simulink model "ModeInputHandle"  (R2018b)
settings: Solver=FixedStepDiscrete  StartTime=0.0  StopTime=10.0  FixedStep=0.01  RelTol=1e-3
undefined symbols (not defined in the file or in its folder): c, CmprtMdHMIReqExt2Tp1, CmprtMdHMIReqExtTp1, CmprtMdHMIReqTp1, d, e, EZESwReq1, f, g, IfVeSMSeStNumConfig, j, KeSMSuButtonLongPressedThrshldTm_Val, KeSMSuFoldType_Val, KeSMSwSeatSMSSeatMdTrigGapTimer_Val, KeSMSwSeatTrigWaitTimer_Val, KeSMSwSRSActiveValidTm_Val, LckUlckActvtFunc1, LstLckFunc1, LugSelectSw1, MdReqTp1, PowerMode1, SeatOccupiedSts1, SRSMode1, StPassCmprtMdCtrl_Md10_VCUConfig_Val, StPassCmprtMdCtrl_Md11_VCUConfig_Val, StPassCmprtMdCtrl_Md12_VCUConfig_Val, StPassCmprtMdCtrl_Md13_VCUConfig_Val, StPassCmprtMdCtrl_Md1_VCUConfig_Val, StPassCmprtMdCtrl_Md27_VCUConfig_Val, StPassCmprtMdCtrl_Md28_VCUConfig_Val, StPassCmprtMdCtrl_Md29_VCUConfig_Val, StPassCmprtMdCtrl_Md2_VCUConfig_Val, StPassCmprtMdCtrl_Md30_VCUConfig_Val, StPassCmprtMdCtrl_Md31_VCUConfig_Val, StPassCmprtMdCtrl_Md32_VCUConfig_Val, StPassCmprtMdCtrl_Md3_VCUConfig_Val, StPassCmprtMdCtrl_Md53_VCUConfig_Val, StPassCmprtMdCtrl_Md56_VCUConfig_Val, StPassCmprtMdCtrl_Md57_VCUConfig_Val, StPassCmprtMdCtrl_Md58_VCUConfig_Val, StPassCmprtMdCtrl_Md61_VCUConfig_Val, StPassCmprtMdCtrl_Md62_VCUConfig_Val, StPassCmprtMdCtrl_Md8_VCUConfig_Val, StPassCmprtMdCtrl_Md9_VCUConfig_Val, StSrv_StMd10_Config_Val, StSrv_StMd11_Config_Val, StSrv_StMd12_Config_Val, StSrv_StMd13_Config_Val, StSrv_StMd1_Config_Val, StSrv_StMd27_Config_Val, StSrv_StMd28_Config_Val, StSrv_StMd29_Config_Val, StSrv_StMd2_Config_Val, StSrv_StMd30_Config_Val, StSrv_StMd31_Config_Val, StSrv_StMd32_Config_Val, StSrv_StMd3_Config_Val, StSrv_StMd8_Config_Val, StSrv_StMd9_Config_Val, VehMovState1
libraries: MSMLib x91
(part 7 of 9)

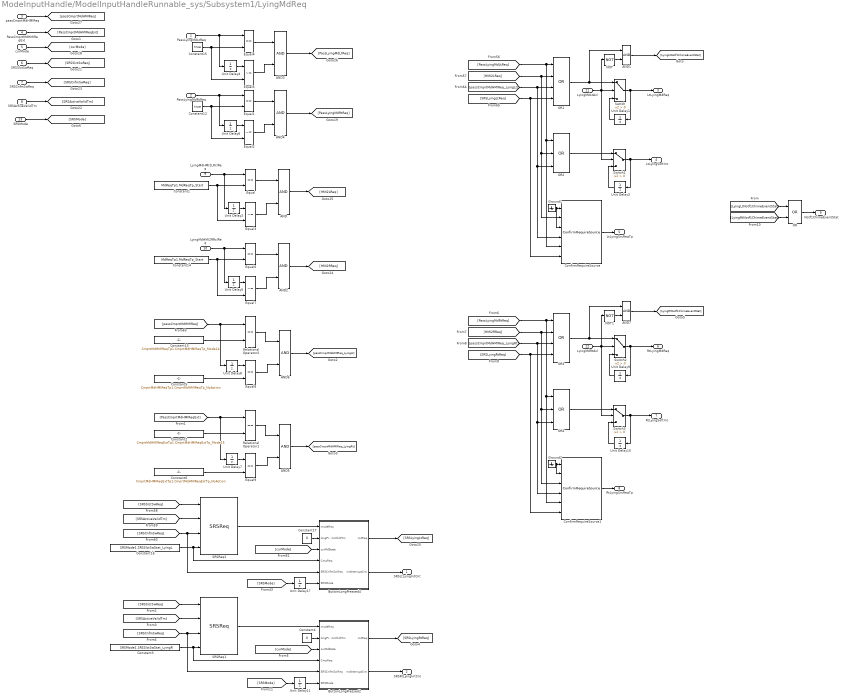
== system ModeInputHandle/ModelInputHandleRunnable_sys/Subsystem1/LyingMdReq ==
  PassLyingMdLtReq : Inport
  PassLyingMdRtReq : Inport  Port=2
  passCmprtMdHMIReq : Inport  Port=3
  PassCmprtMdHMIReqExt : Inport  Port=4
  curMode : Inport  Port=5
  SRSSlctSwReq : Inport  Port=6
  SRSCnfmSwReq : Inport  Port=7
  SRSActiveValidTm : Inport  Port=8
  LyingMdHMI2LRclReq : Inport  Port=9
  LyingMdHMI2RRclReq : Inport  Port=10
  LyingMdLtAvl : Inport  Port=11
  LyingMdRtAvl : Inport  Port=12
  SRSMode : Inport  Port=13
  AND{,1..7} (8 alike) : Logic  AllPortsSameDT=off  OutDataTypeStr=boolean
  ButtonLongPressed2 : Subsystem  AncestorBlock=MSMLib/ButtonLongPressed
  ButtonLongPressed4 : Subsystem  AncestorBlock=MSMLib/ButtonLongPressed
  ConfirmRequireSource : MSMLib/ConfirmRequireSource  SystemSampleTime=-1
  ConfirmRequireSource1 : MSMLib/ConfirmRequireSource  SystemSampleTime=-1
  Constant1 : Constant  Value=MdReqTp1.MdReqTp_Start
  Constant12 : Constant  Value=true  OutDataTypeStr=boolean
  Constant13 : Constant  Value=CmprtMdHMIReqTp1.CmprtMdHMIReqTp_Mode14  OutDataTypeStr=Enum:CmprtMdHMIReqTp1
  Constant14 : Constant  Value=MdReqTp1.MdReqTp_Start
  Constant15 : Constant  Value=true  OutDataTypeStr=boolean
  Constant16 : Constant  Value=SRSMode1.SRSSlctSwStat_LyingL  OutDataTypeStr=Enum:SRSMode1
  Constant17 : Constant  Value=0  OutDataTypeStr=uint8
  Constant2 : Constant  Value=CmprtMdHMIReqExtTp1.CmprtMdHMIReqExtTp_Mode15  OutDataTypeStr=Enum:CmprtMdHMIReqExtTp1
  Constant3 : Constant  Value=SRSMode1.SRSSlctSwStat_LyingR  OutDataTypeStr=Enum:SRSMode1
  Constant4 : Constant  Value=0  OutDataTypeStr=uint8
  Constant5 : Constant  Value=CmprtMdHMIReqTp1.CmprtMdHMIReqTp_NoAction  OutDataTypeStr=Enum:CmprtMdHMIReqTp1
  Constant6 : Constant  Value=CmprtMdHMIReqExtTp1.CmprtMdHMIReqExtTp_NoAction  OutDataTypeStr=Enum:CmprtMdHMIReqExtTp1
  Equal{,1,4,6,8..9} (6 alike) : RelationalOperator  Operator===  OutDataTypeStr=boolean  RndMeth=Simplest
  Equal{2..3,5,7} (4 alike) : RelationalOperator  Operator=~=  OutDataTypeStr=boolean  RndMeth=Simplest
  Ground1 : Ground
  Ground2 : Ground
  NOT : Logic  Operator=NOT  AllPortsSameDT=off  OutDataTypeStr=boolean
  NOT1 : Logic  Operator=NOT  AllPortsSameDT=off  OutDataTypeStr=boolean
  OR : Logic  Operator=OR  AllPortsSameDT=off  OutDataTypeStr=boolean
  OR1 : Logic  Operator=OR  Inputs=4  AllPortsSameDT=off  OutDataTypeStr=boolean
  OR2 : Logic  Operator=OR  Inputs=3  AllPortsSameDT=off  OutDataTypeStr=boolean
  OR3 : Logic  Operator=OR  Inputs=4  AllPortsSameDT=off  OutDataTypeStr=boolean
  OR4 : Logic  Operator=OR  Inputs=3  AllPortsSameDT=off  OutDataTypeStr=boolean
  Relational Operator1 : RelationalOperator  Operator===  OutDataTypeStr=boolean  RndMeth=Simplest
  Relational Operator2 : RelationalOperator  Operator===  OutDataTypeStr=boolean  RndMeth=Simplest
  SRSReq1 : MSMLib/SRSReq  SystemSampleTime=-1
  SRSReq2 : MSMLib/SRSReq  SystemSampleTime=-1
  Switch{,1..3} (4 alike) : Switch  Criteria=u2 > Threshold
  Unit Delay{1,3..4,6,9..10} (6 alike) : UnitDelay  SampleTime=-1
  Unit Delay11 : UnitDelay  InitialCondition=d  SampleTime=-1
  Unit Delay17 : UnitDelay  InitialCondition=d  SampleTime=-1
  Unit Delay2 : UnitDelay  InitialCondition=e  SampleTime=-1
  Unit Delay5 : UnitDelay  InitialCondition=e  SampleTime=-1
  Unit Delay7 : UnitDelay  InitialCondition=g  SampleTime=-1
  Unit Delay8 : UnitDelay  InitialCondition=c  SampleTime=-1
  SRSLtLyingIntCnt : Outport
  SRSRtLyingIntCnt : Outport  Port=2
  LtLyingMdReq : Outport  Port=3
  LtLyingSoftInt : Outport  Port=4
  LtLyingSrcReqTp : Outport  Port=5
  RtLyingMdReq : Outport  Port=6
  RtLyingSoftInt : Outport  Port=7
  RtLyingSrcReqTp : Outport  Port=8
  Notf1ChimeEventStat : Outport  Port=9
  wires:
  Constant15/1 -> Equal4/2, Equal5/2
  Equal5/1 -> AND3/2
  PassLyingMdLtReq/1 -> Unit Delay4/1, Equal4/1
  Equal2/1 -> AND4/2
  Constant12/1 -> Equal1/2, Equal2/2
  AND4/1 -> [PassLyingMdRtReq]
  Unit Delay4/1 -> Equal5/1
  Equal1/1 -> AND4/1
  PassLyingMdRtReq/1 -> Unit Delay6/1, Equal1/1
  Equal4/1 -> AND3/1
  AND3/1 -> [PassLyingMdLtReq]
  Unit Delay6/1 -> Equal2/1
  passCmprtMdHMIReq/1 -> [passCmprtMdHMIReq]
  SRSActiveValidTm/1 -> [SRSActiveValidTm]
  SRSSlctSwReq/1 -> [SRSSlctSwReq]
  SRSCnfmSwReq/1 -> [SRSCnfmSwReq]
  curMode/1 -> [curMode]
  PassCmprtMdHMIReqExt/1 -> [PassCmprtMdHMIReqExt]
  AND/1 -> [HMI2LReq]
  Equal3/1 -> AND/2
  Equal/1 -> AND/1
  Equal6/1 -> AND2/1
  Constant1/1 -> Equal3/2, Equal/2
  Constant14/1 -> Equal7/2, Equal6/2
  AND2/1 -> [HMI2RReq]
  Equal7/1 -> AND2/2
  Unit Delay5/1 -> Equal7/1
  LyingMdHMI2RRclReq/1 -> Unit Delay5/1, Equal6/1
  Unit Delay2/1 -> Equal3/1
  LyingMdHMI2LRclReq/1 -> Unit Delay2/1, Equal/1
  Unit Delay7/1 -> Equal9/1
  AND5/1 -> [passCmprtMdHMIReq_LyingRt]
  Equal9/1 -> AND5/2
  [PassCmprtMdHMIReqExt] -> Unit Delay7/1, Relational Operator1/1
  Constant2/1 -> Relational Operator1/2
  Relational Operator1/1 -> AND5/1
  [passCmprtMdHMIReq] -> Unit Delay8/1, Relational Operator2/1
  Relational Operator2/1 -> AND6/1
  Equal8/1 -> AND6/2
  Constant13/1 -> Relational Operator2/2
  Unit Delay8/1 -> Equal8/1
  AND6/1 -> [passCmprtMdHMIReq_LyingLt]
  Constant3/1 -> ButtonLongPressed2/4(CmpReq), SRSReq1/4
  ButtonLongPressed2/1(mdReq) -> [SRSLyingRtReq]
  [SRSCnfmSwReq] -> ButtonLongPressed2/5(SRSCnfmSwReq), SRSReq1/3
  Constant4/1 -> ButtonLongPressed2/2(longPressThrshhldTm)
  [SRSSlctSwReq] -> SRSReq1/1
  ButtonLongPressed2/2(mdInterruptCnt) -> SRSRtLyingIntCnt/1
  SRSReq1/1 -> ButtonLongPressed2/1(modeReq)
  SRSReq2/1 -> ButtonLongPressed4/1(modeReq)
  [SRSActiveValidTm] -> SRSReq1/2
  [SRSSlctSwReq] -> SRSReq2/1
  [curMode] -> ButtonLongPressed4/3(curMdState)
  Constant17/1 -> ButtonLongPressed4/2(longPressThrshhldTm)
  [curMode] -> ButtonLongPressed2/3(curMdState)
  [SRSActiveValidTm] -> SRSReq2/2
  Constant16/1 -> ButtonLongPressed4/4(CmpReq), SRSReq2/4
  ButtonLongPressed4/1(mdReq) -> [SRSLyingLtReq]
  [SRSCnfmSwReq] -> ButtonLongPressed4/5(SRSCnfmSwReq), SRSReq2/3
  ButtonLongPressed4/2(mdInterruptCnt) -> SRSLtLyingIntCnt/1
  Switch1/1 -> LtLyingSoftInt/1, Unit Delay3/1
  Unit Delay3/1 -> Switch1/3
  NOT/1 -> AND1/2
  OR1/1 -> AND1/1, Switch/1
  [PassLyingMdLtReq] -> ConfirmRequireSource/5, OR2/1, OR1/1
  [passCmprtMdHMIReq_LyingLt] -> ConfirmRequireSource/4, OR2/3, OR1/3
  Ground1/1 -> ConfirmRequireSource/3, ConfirmRequireSource/1
  ConfirmRequireSource/1 -> LtLyingSrcReqTp/1
  [SRSLyingLtReq] -> ConfirmRequireSource/6, OR1/4
  Switch/1 -> LtLyingMdReq/1, Unit Delay1/1
  OR2/1 -> Switch1/1
  LyingMdLtAvl/1 -> Switch1/2, NOT/1, Switch/2
  Unit Delay1/1 -> Switch/3
  AND1/1 -> [LyingLtNotf1ChimeEventStat]
  [HMI2LReq] -> ConfirmRequireSource/2, OR2/2, OR1/2
  AND7/1 -> [LyingRtNotf1ChimeEventStat]
  Unit Delay9/1 -> Switch2/3
  OR4/1 -> Switch3/1
  [PassLyingMdRtReq] -> ConfirmRequireSource1/5, OR4/1, OR3/1
  LyingMdRtAvl/1 -> Switch3/2, NOT1/1, Switch2/2
  Switch2/1 -> RtLyingMdReq/1, Unit Delay9/1
  [SRSLyingRtReq] -> ConfirmRequireSource1/6, OR3/4
  [passCmprtMdHMIReq_LyingRt] -> ConfirmRequireSource1/4, OR4/3, OR3/3
  ConfirmRequireSource1/1 -> RtLyingSrcReqTp/1
  Ground2/1 -> ConfirmRequireSource1/2, ConfirmRequireSource1/1
  [HMI2RReq] -> ConfirmRequireSource1/3, OR4/2, OR3/2
  OR3/1 -> AND7/1, Switch2/1
  NOT1/1 -> AND7/2
  Switch3/1 -> RtLyingSoftInt/1, Unit Delay10/1
  Unit Delay10/1 -> Switch3/3
  [LyingLtNotf1ChimeEventStat] -> OR/1
  OR/1 -> Notf1ChimeEventStat/1
  [LyingRtNotf1ChimeEventStat] -> OR/2
  Unit Delay17/1 -> ButtonLongPressed4/6(SRSMode)
  [SRSMode] -> Unit Delay17/1
  Unit Delay11/1 -> ButtonLongPressed2/6(SRSMode)
  [SRSMode] -> Unit Delay11/1
  SRSMode/1 -> [SRSMode]
  Constant5/1 -> Equal8/2
  Constant6/1 -> Equal9/2

== system ModeInputHandle/ModelInputHandleRunnable_sys/Subsystem1/PasReclinerEntryMdReq ==
  PassStFldDnMovSwAct : Inport
  PassStFldDnMovSwActV : Inport  Port=2
  buttonLongPressedThrshhldTm : Inport  Port=3
  PassCmprtMdHMIReqExt : Inport  Port=4
  PassPasReclinerEntryReq : Inport  Port=5
  PasReclinerAvl : Inport  Port=6
  StPassCmprtMdCtrl_Md30_VCUConfig : Inport  Port=7
  StSrv_StMd30_Config : Inport  Port=8
  AND : Logic  AllPortsSameDT=off  OutDataTypeStr=boolean
  AND2 : Logic  AllPortsSameDT=off  OutDataTypeStr=boolean
  AND5 : Logic  AllPortsSameDT=off  OutDataTypeStr=boolean
  ButtonLongPressed : Subsystem  AncestorBlock=MSMLib/ButtonLongPressed
  ConfirmRequireSource : MSMLib/ConfirmRequireSource  SystemSampleTime=-1
  Constant : Constant  Value=0  OutDataTypeStr=boolean
  Constant1 : Constant  Value=0  OutDataTypeStr=boolean
  Constant19 : Constant  Value=7  OutDataTypeStr=uint8
  Constant2 : Constant  Value=CmprtMdHMIReqExtTp1.CmprtMdHMIReqExtTp_Mode30  OutDataTypeStr=Enum:CmprtMdHMIReqExtTp1
  Constant3 : Constant  Value=CmprtMdHMIReqExtTp1.CmprtMdHMIReqExtTp_NoAction  OutDataTypeStr=Enum:CmprtMdHMIReqExtTp1
  Constant4 : Constant  Value=true  OutDataTypeStr=boolean
  Equal17 : RelationalOperator  Operator=~=  OutDataTypeStr=boolean  RndMeth=Simplest
  Equal2 : RelationalOperator  Operator===  OutDataTypeStr=boolean  RndMeth=Simplest
  Equal4 : RelationalOperator  Operator===  OutDataTypeStr=boolean  RndMeth=Simplest
  Equal5 : RelationalOperator  Operator=~=  OutDataTypeStr=boolean  RndMeth=Simplest
  Ground : Ground
  Logical Operator : Logic  Operator=OR  Inputs=3  AllPortsSameDT=off  OutDataTypeStr=boolean
  NOT : Logic  Operator=NOT  AllPortsSameDT=off  OutDataTypeStr=boolean
  OR1 : Logic  Operator=OR  AllPortsSameDT=off  OutDataTypeStr=boolean
  Relational Operator3 : RelationalOperator  Operator===  OutDataTypeStr=boolean  RndMeth=Simplest
  SWIntSrc_S : MSMLib/SWIntSrc_S  SystemSampleTime=-1
  Subsystem4 : MSMLib/MergeReqAndValidity  SystemSampleTime=-1
  Switch{,1..3} (4 alike) : Switch  Criteria=u2 > Threshold
  Unit Delay{,1..2,19} (4 alike) : UnitDelay  SampleTime=-1
  Unit Delay3 : UnitDelay  InitialCondition=g  SampleTime=-1
  SwPasReclinerEntryIntCnt : Outport
  PasReclinerEntryReq : Outport  Port=2  VectorParamsAs1DForOutWhenUnconnected=on
  srcReqTp : Outport  Port=3  VectorParamsAs1DForOutWhenUnconnected=on
  PasReclinerEntrySoftInt : Outport  Port=4
  Notf1ChimeEventStat : Outport  Port=5
  wires:
  Subsystem4/1 -> ButtonLongPressed/1(modeReq)
  PassStFldDnMovSwAct/1 -> Subsystem4/1
  ButtonLongPressed/2(mdInterruptCnt) -> SwPasReclinerEntryIntCnt/1, Unit Delay19/1, Equal17/1
  buttonLongPressedThrshhldTm/1 -> ButtonLongPressed/2(longPressThrshhldTm)
  Constant19/1 -> SWIntSrc_S/2
  Equal17/1 -> SWIntSrc_S/1
  ButtonLongPressed/1(mdReq) -> [SwPasReclinerEntryMdReq]
  PassStFldDnMovSwActV/1 -> Subsystem4/2
  Unit Delay19/1 -> Equal17/2
  Unit Delay2/1 -> Equal5/1
  Equal5/1 -> AND2/2
  PassPasReclinerEntryReq/1 -> Unit Delay2/1, Equal4/1
  Constant4/1 -> Equal4/2, Equal5/2
  Equal4/1 -> AND2/1
  Logical Operator/1 -> Switch1/1, AND/1
  Unit Delay1/1 -> Switch2/3
  OR1/1 -> Switch2/1
  NOT/1 -> AND/2
  Unit Delay/1 -> Switch1/3
  PasReclinerAvl/1 -> Switch2/2, NOT/1, Switch1/2
  Switch2/1 -> PasReclinerEntrySoftInt/1, Unit Delay1/1
  [PassPasReclinerEntryReq] -> ConfirmRequireSource/5, OR1/1, Logical Operator/2
  [SwPasReclinerEntryMdReq] -> ConfirmRequireSource/1, Logical Operator/1
  Switch1/1 -> Unit Delay/1, PasReclinerEntryReq/1
  [passCmprtMdHMIReq_PasReclinerEntry] -> ConfirmRequireSource/4, OR1/2, Logical Operator/3
  ConfirmRequireSource/1 -> srcReqTp/1
  AND/1 -> Notf1ChimeEventStat/1
  Ground/1 -> ConfirmRequireSource/6, ConfirmRequireSource/3, ConfirmRequireSource/2
  PassCmprtMdHMIReqExt/1 -> Relational Operator3/1, Unit Delay3/1
  Unit Delay3/1 -> Equal2/1
  Constant3/1 -> Equal2/2
  Relational Operator3/1 -> AND5/1
  Constant2/1 -> Relational Operator3/2
  Equal2/1 -> AND5/2
  StPassCmprtMdCtrl_Md30_VCUConfig/1 -> Switch/2
  AND5/1 -> Switch/1
  Constant/1 -> Switch/3
  Switch/1 -> [passCmprtMdHMIReq_PasReclinerEntry]
  AND2/1 -> Switch3/1
  StSrv_StMd30_Config/1 -> Switch3/2
  Constant1/1 -> Switch3/3
  Switch3/1 -> [PassPasReclinerEntryReq]

== system ModeInputHandle/ModelInputHandleRunnable_sys/Subsystem1/PasReclinerExitMdReq ==
  PassStFldUpMovSwAct : Inport
  PassStFldUpMovSwActV : Inport  Port=2
  buttonLongPressedThrshhldTm : Inport  Port=3
  PassCmprtMdHMIReqExt : Inport  Port=4
  PassPasReclinerExitReq : Inport  Port=5
  PasReclinerExitAvl : Inport  Port=6
  StPassCmprtMdCtrl_Md31_VCUConfig : Inport  Port=7
  StSrv_StMd31_Config : Inport  Port=8
  AND : Logic  AllPortsSameDT=off  OutDataTypeStr=boolean
  AND2 : Logic  AllPortsSameDT=off  OutDataTypeStr=boolean
  AND5 : Logic  AllPortsSameDT=off  OutDataTypeStr=boolean
  ButtonLongPressed : Subsystem  AncestorBlock=MSMLib/ButtonLongPressed
  ConfirmRequireSource : MSMLib/ConfirmRequireSource  SystemSampleTime=-1
  Constant : Constant  Value=0  OutDataTypeStr=boolean
  Constant1 : Constant  Value=0  OutDataTypeStr=boolean
  Constant19 : Constant  Value=8  OutDataTypeStr=uint8
  Constant2 : Constant  Value=CmprtMdHMIReqExtTp1.CmprtMdHMIReqExtTp_Mode31  OutDataTypeStr=Enum:CmprtMdHMIReqExtTp1
  Constant3 : Constant  Value=CmprtMdHMIReqExtTp1.CmprtMdHMIReqExtTp_NoAction  OutDataTypeStr=Enum:CmprtMdHMIReqExtTp1
  Constant4 : Constant  Value=true  OutDataTypeStr=boolean
  Equal17 : RelationalOperator  Operator=~=  OutDataTypeStr=boolean  RndMeth=Simplest
  Equal2 : RelationalOperator  Operator===  OutDataTypeStr=boolean  RndMeth=Simplest
  Equal4 : RelationalOperator  Operator===  OutDataTypeStr=boolean  RndMeth=Simplest
  Equal5 : RelationalOperator  Operator=~=  OutDataTypeStr=boolean  RndMeth=Simplest
  Ground : Ground
  Logical Operator : Logic  Operator=OR  Inputs=3  AllPortsSameDT=off  OutDataTypeStr=boolean
  NOT : Logic  Operator=NOT  AllPortsSameDT=off  OutDataTypeStr=boolean
  OR1 : Logic  Operator=OR  AllPortsSameDT=off  OutDataTypeStr=boolean
  Relational Operator3 : RelationalOperator  Operator===  OutDataTypeStr=boolean  RndMeth=Simplest
  SWIntSrc_S : MSMLib/SWIntSrc_S  SystemSampleTime=-1
  Subsystem4 : MSMLib/MergeReqAndValidity  SystemSampleTime=-1
  Switch{,1..3} (4 alike) : Switch  Criteria=u2 > Threshold
  Unit Delay{,1..2,19} (4 alike) : UnitDelay  SampleTime=-1
  Unit Delay3 : UnitDelay  InitialCondition=g  SampleTime=-1
  SwPasReclinerExitIntCnt : Outport
  PasReclinerExitReq : Outport  Port=2  VectorParamsAs1DForOutWhenUnconnected=on
  srcReqTp : Outport  Port=3  VectorParamsAs1DForOutWhenUnconnected=on
  PasReclinerExitSoftInt : Outport  Port=4
  Notf1ChimeEventStat : Outport  Port=5
  wires:
  Ground/1 -> ConfirmRequireSource/2, ConfirmRequireSource/3, ConfirmRequireSource/6
  AND/1 -> Notf1ChimeEventStat/1
  ConfirmRequireSource/1 -> srcReqTp/1
  [passCmprtMdHMIReq_PasReclinerExit] -> Logical Operator/3, OR1/2, ConfirmRequireSource/4
  Switch1/1 -> PasReclinerExitReq/1, Unit Delay/1
  [SwPasReclinerExitMdReq] -> Logical Operator/1, ConfirmRequireSource/1
  [PassPasReclinerExitReq] -> Logical Operator/2, OR1/1, ConfirmRequireSource/5
  Switch2/1 -> Unit Delay1/1, PasReclinerExitSoftInt/1
  PasReclinerExitAvl/1 -> Switch1/2, NOT/1, Switch2/2
  Unit Delay/1 -> Switch1/3
  NOT/1 -> AND/2
  OR1/1 -> Switch2/1
  Unit Delay1/1 -> Switch2/3
  Logical Operator/1 -> AND/1, Switch1/1
  Equal4/1 -> AND2/1
  Constant4/1 -> Equal5/2, Equal4/2
  PassPasReclinerExitReq/1 -> Equal4/1, Unit Delay2/1
  Equal5/1 -> AND2/2
  Unit Delay2/1 -> Equal5/1
  Unit Delay19/1 -> Equal17/2
  PassStFldUpMovSwActV/1 -> Subsystem4/2
  ButtonLongPressed/1(mdReq) -> [SwPasReclinerExitMdReq]
  Equal17/1 -> SWIntSrc_S/1
  Constant19/1 -> SWIntSrc_S/2
  buttonLongPressedThrshhldTm/1 -> ButtonLongPressed/2(longPressThrshhldTm)
  ButtonLongPressed/2(mdInterruptCnt) -> Equal17/1, Unit Delay19/1, SwPasReclinerExitIntCnt/1
  PassStFldUpMovSwAct/1 -> Subsystem4/1
  Subsystem4/1 -> ButtonLongPressed/1(modeReq)
  PassCmprtMdHMIReqExt/1 -> Relational Operator3/1, Unit Delay3/1
  Relational Operator3/1 -> AND5/1
  Unit Delay3/1 -> Equal2/1
  Constant2/1 -> Relational Operator3/2
  Constant3/1 -> Equal2/2
  Equal2/1 -> AND5/2
  StPassCmprtMdCtrl_Md31_VCUConfig/1 -> Switch/2
  AND5/1 -> Switch/1
  Constant/1 -> Switch/3
  Switch/1 -> [passCmprtMdHMIReq_PasReclinerExit]
  AND2/1 -> Switch3/1
  StSrv_StMd31_Config/1 -> Switch3/2
  Switch3/1 -> [PassPasReclinerExitReq]
  Constant1/1 -> Switch3/3

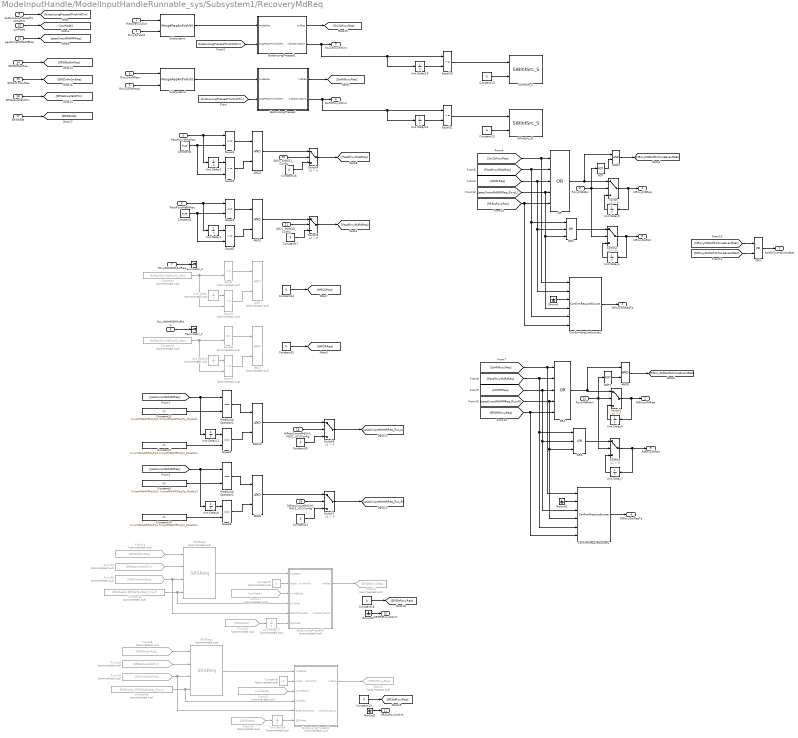
== system ModeInputHandle/ModelInputHandleRunnable_sys/Subsystem1/RecoveryMdReq ==
  Recovery2LSwt : Inport
  RcvySwValid : Inport  Port=2
  RcvySwRtReq : Inport  Port=3
  RcvySwRtReqV : Inport  Port=4
  PassRcvyMdLtReq : Inport  Port=5
  PassRcvyMdRtReq : Inport  Port=6
  RcvyMdHMI2LRclReq : Inport  Port=7
  RcvyMdHMI2RRclReq : Inport  Port=8
  buttonLongPressedThrshhldTm : Inport  Port=9
  curMode : Inport  Port=10
  RcvyMdLtAvl : Inport  Port=11
  RcvyMdRtAvl : Inport  Port=12
  passCmprtMdHMIReq : Inport  Port=13
  SRSSlctSwReq : Inport  Port=14
  SRSCnfmSwReq : Inport  Port=15
  SRSActiveValidTm : Inport  Port=16
  SRSMode : Inport  Port=17
  StPassCmprtMdCtrl_Md11_VCUConfig : Inport  Port=18
  StPassCmprtMdCtrl_Md13_VCUConfig : Inport  Port=19
  StSrv_StMd11_Config : Inport  Port=20
  StSrv_StMd13_Config : Inport  Port=21
  AND : Logic  Commented=on  AllPortsSameDT=off  OutDataTypeStr=boolean
  AND{1,3..6,10} (6 alike) : Logic  AllPortsSameDT=off  OutDataTypeStr=boolean
  AND2 : Logic  Commented=on  AllPortsSameDT=off  OutDataTypeStr=boolean
  ButtonLongPressed : Subsystem  AncestorBlock=MSMLib/ButtonLongPressed
  ButtonLongPressed1 : Subsystem  AncestorBlock=MSMLib/ButtonLongPressed
  ButtonLongPressed2 : Subsystem  Commented=on  AncestorBlock=MSMLib/ButtonLongPressed
  ButtonLongPressed4 : Subsystem  Commented=on  AncestorBlock=MSMLib/ButtonLongPressed
  ConfirmRequireSource1 : MSMLib/ConfirmRequireSource  SystemSampleTime=-1
  ConfirmRequireSource2 : MSMLib/ConfirmRequireSource  SystemSampleTime=-1
  Constant : Constant  Commented=on  Value=MdReqTp1.MdReqTp_Start
  Constant1 : Constant  Value=true  OutDataTypeStr=boolean
  Constant10 : Constant  Value=CmprtMdHMIReqTp1.CmprtMdHMIReqTp_NoAction  OutDataTypeStr=Enum:CmprtMdHMIReqTp1
  Constant11 : Constant  Value=CmprtMdHMIReqTp1.CmprtMdHMIReqTp_Mode11  OutDataTypeStr=Enum:CmprtMdHMIReqTp1
  Constant12 : Constant  Value=5  OutDataTypeStr=uint8
  Constant13 : Constant  Value=6  OutDataTypeStr=uint8
  Constant{14..21} (8 alike) : Constant  Value=0  OutDataTypeStr=boolean
  Constant2 : Constant  Commented=on  Value=MdReqTp1.MdReqTp_Start
  Constant3 : Constant  Value=CmprtMdHMIReqTp1.CmprtMdHMIReqTp_Mode13  OutDataTypeStr=Enum:CmprtMdHMIReqTp1
  Constant4 : Constant  Value=true  OutDataTypeStr=boolean
  Constant5 : Constant  Commented=on  Value=SRSMode1.SRSSlctSwStat_RcvyL  OutDataTypeStr=Enum:SRSMode1
  Constant6 : Constant  Commented=on  Value=0  OutDataTypeStr=uint8
  Constant7 : Constant  Value=CmprtMdHMIReqTp1.CmprtMdHMIReqTp_NoAction  OutDataTypeStr=Enum:CmprtMdHMIReqTp1
  Constant8 : Constant  Commented=on  Value=SRSMode1.SRSSlctSwStat_RcvyR  OutDataTypeStr=Enum:SRSMode1
  Constant9 : Constant  Commented=on  Value=0  OutDataTypeStr=uint8
  Equal : RelationalOperator  Commented=on  Operator===  OutDataTypeStr=boolean  RndMeth=Simplest
  Equal{1,4,8..9} (4 alike) : RelationalOperator  Operator===  OutDataTypeStr=boolean  RndMeth=Simplest
  Equal{2,5,10..11} (4 alike) : RelationalOperator  Operator=~=  OutDataTypeStr=boolean  RndMeth=Simplest
  Equal3 : RelationalOperator  Commented=on  Operator=~=  OutDataTypeStr=boolean  RndMeth=Simplest
  Equal6 : RelationalOperator  Commented=on  Operator===  OutDataTypeStr=boolean  RndMeth=Simplest
  Equal7 : RelationalOperator  Commented=on  Operator=~=  OutDataTypeStr=boolean  RndMeth=Simplest
  From14 : From  Commented=on  GotoTag=SRSSlctSwReq
  From15 : From  Commented=on  GotoTag=SRSActiveValidTm
  From16 : From  Commented=on  GotoTag=SRSCnfmSwReq
  From17 : From  Commented=on  GotoTag=curMode
  From18 : From  Commented=on  GotoTag=SRSSlctSwReq
  From19 : From  Commented=on  GotoTag=SRSActiveValidTm
  From20 : From  Commented=on  GotoTag=SRSCnfmSwReq
  From21 : From  Commented=on  GotoTag=curMode
  From24 : From  Commented=on  GotoTag=SRSMode
  From43 : From  Commented=on  GotoTag=SRSMode
  Goto11 : Goto  Commented=on  GotoTag=SRSRtRcvyReq
  Goto12 : Goto  Commented=on  GotoTag=SRSLtRcvyReq
  Ground{,1..3} (4 alike) : Ground
  NOT : Logic  Operator=NOT  AllPortsSameDT=off  OutDataTypeStr=boolean
  NOT1 : Logic  Operator=NOT  AllPortsSameDT=off  OutDataTypeStr=boolean
  OR : Logic  Operator=OR  Inputs=5  AllPortsSameDT=off  OutDataTypeStr=boolean
  OR1 : Logic  Operator=OR  Inputs=5  AllPortsSameDT=off  OutDataTypeStr=boolean
  OR2 : Logic  Operator=OR  AllPortsSameDT=off  OutDataTypeStr=boolean
  OR3 : Logic  Operator=OR  Inputs=3  AllPortsSameDT=off  OutDataTypeStr=boolean
  OR4 : Logic  Operator=OR  Inputs=3  AllPortsSameDT=off  OutDataTypeStr=boolean
  Relational Operator1 : RelationalOperator  Operator===  OutDataTypeStr=boolean  RndMeth=Simplest
  Relational Operator2 : RelationalOperator  Operator===  OutDataTypeStr=boolean  RndMeth=Simplest
  SRSReq1 : MSMLib/SRSReq  Commented=on  SystemSampleTime=-1
  SRSReq2 : MSMLib/SRSReq  Commented=on  SystemSampleTime=-1
  SWIntSrc_S : MSMLib/SWIntSrc_S  SystemSampleTime=-1
  SWIntSrc_S1 : MSMLib/SWIntSrc_S  SystemSampleTime=-1
  Subsystem1 : MSMLib/MergeReqAndValidity  SystemSampleTime=-1
  Subsystem4 : MSMLib/MergeReqAndValidity  SystemSampleTime=-1
  Switch{,1..7} (8 alike) : Switch  Criteria=u2 > Threshold
  Terminator_1 : Terminator
  Terminator_2 : Terminator
  Unit Delay : UnitDelay  Commented=on  InitialCondition=e  SampleTime=-1
  Unit Delay{1..2,4..7,10,12} (8 alike) : UnitDelay  SampleTime=-1
  Unit Delay11 : UnitDelay  InitialCondition=c  SampleTime=-1
  Unit Delay17 : UnitDelay  Commented=on  InitialCondition=d  SampleTime=-1
  Unit Delay3 : UnitDelay  Commented=on  InitialCondition=e  SampleTime=-1
  Unit Delay8 : UnitDelay  InitialCondition=c  SampleTime=-1
  Unit Delay9 : UnitDelay  Commented=on  InitialCondition=d  SampleTime=-1
  LtRcvyMdReq : Outport
  RtRcvyMdReq : Outport  Port=2
  LtRcvySrcReqTp : Outport  Port=3
  RtRcvySrcReqTp : Outport  Port=4
  Sw2LRcvyIntCnt : Outport  Port=5
  SwRtRcvyIntCnt : Outport  Port=6
  Notf1ChimeEventStat : Outport  Port=7
  LtRcvySoftInt : Outport  Port=8
  RtRcvySoftInt : Outport  Port=9
  SRSRtRcvyIntCnt : Outport  Port=10
  SRSLtRcvyIntCnt : Outport  Port=11
  wires:
  curMode/1 -> [curMode]
  buttonLongPressedThrshhldTm/1 -> [buttonLongPressedThrshhldTm]
  ButtonLongPressed1/2(mdInterruptCnt) -> Unit Delay10/1, Equal10/1, Sw2LRcvyIntCnt/1
  [buttonLongPressedThrshhldTm] -> ButtonLongPressed1/2(longPressThrshhldTm)
  ButtonLongPressed1/1(mdReq) -> [Sw2LRcvyReq]
  RcvySwRtReq/1 -> Subsystem4/1
  Subsystem4/1 -> ButtonLongPressed/1(modeReq)
  ButtonLongPressed/1(mdReq) -> [SwRtRcvyReq]
  [buttonLongPressedThrshhldTm] -> ButtonLongPressed/2(longPressThrshhldTm)
  RcvySwRtReqV/1 -> Subsystem4/2
  ButtonLongPressed/2(mdInterruptCnt) -> Unit Delay12/1, Equal11/1, SwRtRcvyIntCnt/1
  Equal4/1 -> AND3/1
  Equal5/1 -> AND3/2
  Unit Delay2/1 -> Equal5/1
  PassRcvyMdLtReq/1 -> Unit Delay2/1, Equal4/1
  Constant4/1 -> Equal4/2, Equal5/2
  Constant1/1 -> Equal1/2, Equal2/2
  Equal1/1 -> AND1/1
  PassRcvyMdRtReq/1 -> Unit Delay1/1, Equal1/1
  Unit Delay1/1 -> Equal2/1
  Equal2/1 -> AND1/2
  Unit Delay/1 -> Equal3/1
  Constant/1 -> Equal3/2, Equal/2
  Equal/1 -> AND/1
  Equal3/1 -> AND/2
  Unit Delay3/1 -> Equal7/1
  Equal7/1 -> AND2/2
  Constant2/1 -> Equal7/2, Equal6/2
  Equal6/1 -> AND2/1
  [Sw2LRcvyReq] -> ConfirmRequireSource1/1, OR/1
  [PassRcvyMdLtReq] -> OR/2, ConfirmRequireSource1/5, OR3/1
  [HMI2LReq] -> OR3/2, ConfirmRequireSource1/2, OR/3
  Unit Delay5/1 -> Switch/3
  Switch/1 -> LtRcvyMdReq/1, Unit Delay5/1
  RcvyMdLtAvl/1 -> Switch2/2, NOT/1, Switch/2
  OR/1 -> AND4/1, Switch/1
  [PassRcvyMdRtReq] -> ConfirmRequireSource2/5, OR4/1, OR1/2
  [HMI2RReq] -> ConfirmRequireSource2/3, OR4/2, OR1/3
  OR1/1 -> Switch1/1, AND5/1
  Unit Delay4/1 -> Switch1/3
  Switch1/1 -> RtRcvyMdReq/1, Unit Delay4/1
  RcvyMdRtAvl/1 -> Switch3/2, NOT1/1, Switch1/2
  [SwRtRcvyReq] -> ConfirmRequireSource2/1, OR1/1
  ConfirmRequireSource1/1 -> LtRcvySrcReqTp/1
  ConfirmRequireSource2/1 -> RtRcvySrcReqTp/1
  NOT/1 -> AND4/2
  AND4/1 -> [LtRcvyMdNotf1ChimeEventStat]
  NOT1/1 -> AND5/2
  AND5/1 -> [RtRcvyMdNotf1ChimeEventStat]
  [LtRcvyMdNotf1ChimeEventStat] -> OR2/1
  [RtRcvyMdNotf1ChimeEventStat] -> OR2/2
  OR2/1 -> Notf1ChimeEventStat/1
  OR3/1 -> Switch2/1
  Unit Delay6/1 -> Switch2/3
  Switch2/1 -> Unit Delay6/1, LtRcvySoftInt/1
  OR4/1 -> Switch3/1
  Switch3/1 -> Unit Delay7/1, RtRcvySoftInt/1
  Unit Delay7/1 -> Switch3/3
  Ground/1 -> ConfirmRequireSource1/3
  Ground1/1 -> ConfirmRequireSource2/2
  passCmprtMdHMIReq/1 -> [passCmprtMdHMIReq]
  Relational Operator1/1 -> AND10/1
  [passCmprtMdHMIReq] -> Unit Delay11/1, Relational Operator1/1
  Unit Delay11/1 -> Equal9/1
  Equal9/1 -> AND10/2
  Constant11/1 -> Relational Operator1/2
  [passCmprtMdHMIReq] -> Unit Delay8/1, Relational Operator2/1
  Unit Delay8/1 -> Equal8/1
  Constant3/1 -> Relational Operator2/2
  Equal8/1 -> AND6/2
  Relational Operator2/1 -> AND6/1
  [passCmprtMdHMIReq_RcvyL] -> ConfirmRequireSource1/4, OR3/3, OR/4
  [passCmprtMdHMIReq_RcvyR] -> ConfirmRequireSource2/4, OR4/3, OR1/4
  From14/1 -> SRSReq2/1
  From16/1 -> ButtonLongPressed4/5(SRSCnfmSwReq), SRSReq2/3
  From15/1 -> SRSReq2/2
  SRSReq2/1 -> ButtonLongPressed4/1(modeReq)
  ButtonLongPressed4/1(mdReq) -> Goto11/1
  Constant8/1 -> ButtonLongPressed4/4(CmpReq), SRSReq2/4
  Constant9/1 -> ButtonLongPressed4/2(longPressThrshhldTm)
  From17/1 -> ButtonLongPressed4/3(curMdState)
  SRSSlctSwReq/1 -> [SRSSlctSwReq]
  SRSCnfmSwReq/1 -> [SRSCnfmSwReq]
  SRSActiveValidTm/1 -> [SRSActiveValidTm]
  From20/1 -> ButtonLongPressed2/5(SRSCnfmSwReq), SRSReq1/3
  SRSReq1/1 -> ButtonLongPressed2/1(modeReq)
  Constant6/1 -> ButtonLongPressed2/2(longPressThrshhldTm)
  From21/1 -> ButtonLongPressed2/3(curMdState)
  Constant5/1 -> ButtonLongPressed2/4(CmpReq), SRSReq1/4
  From18/1 -> SRSReq1/1
  From19/1 -> SRSReq1/2
  ButtonLongPressed2/1(mdReq) -> Goto12/1
  [SRSRtRcvyReq] -> ConfirmRequireSource2/6, OR1/5
  [SRSLtRcvyReq] -> ConfirmRequireSource1/6, OR/5
  Subsystem1/1 -> ButtonLongPressed1/1(modeReq)
  Recovery2LSwt/1 -> Subsystem1/1
  RcvySwValid/1 -> Subsystem1/2
  From43/1 -> Unit Delay17/1
  Unit Delay17/1 -> ButtonLongPressed4/6(SRSMode)
  Unit Delay9/1 -> ButtonLongPressed2/6(SRSMode)
  From24/1 -> Unit Delay9/1
  SRSMode/1 -> [SRSMode]
  Constant7/1 -> Equal9/2
  Constant10/1 -> Equal8/2
  Unit Delay10/1 -> Equal10/2
  Equal10/1 -> SWIntSrc_S/1
  Constant12/1 -> SWIntSrc_S/2
  Unit Delay12/1 -> Equal11/2
  Equal11/1 -> SWIntSrc_S1/1
  Constant13/1 -> SWIntSrc_S1/2
  Constant14/1 -> [HMI2LReq]
  Constant15/1 -> [HMI2RReq]
  RcvyMdHMI2LRclReq/1 -> Terminator_2/1
  RcvyMdHMI2RRclReq/1 -> Terminator_1/1
  Constant18/1 -> [SRSRtRcvyReq]
  Constant19/1 -> [SRSLtRcvyReq]
  Ground2/1 -> SRSLtRcvyIntCnt/1
  Ground3/1 -> SRSRtRcvyIntCnt/1
  StSrv_StMd11_Config/1 -> Switch4/2
  AND3/1 -> Switch4/1
  Constant16/1 -> Switch4/3
  Switch4/1 -> [PassRcvyMdLtReq]
  AND1/1 -> Switch5/1
  StSrv_StMd13_Config/1 -> Switch5/2
  Constant17/1 -> Switch5/3
  Switch5/1 -> [PassRcvyMdRtReq]
  StPassCmprtMdCtrl_Md11_VCUConfig/1 -> Switch6/2
  AND10/1 -> Switch6/1
  Constant20/1 -> Switch6/3
  Switch6/1 -> [passCmprtMdHMIReq_RcvyL]
  AND6/1 -> Switch7/1
  StPassCmprtMdCtrl_Md13_VCUConfig/1 -> Switch7/2
  Constant21/1 -> Switch7/3
  Switch7/1 -> [passCmprtMdHMIReq_RcvyR]

== system ModeInputHandle/ModelInputHandleRunnable_sys/Subsystem1/UnfoldMdReq ==
  ThdRLtStExpdSwReq : Inport
  ThdRLtStExpdSwReqV : Inport  Port=2
  ThdRRtStExpdSwReq : Inport  Port=3
  ThdRRtStExpdSwReqV : Inport  Port=4
  buttonLongPressedThrshhldTm : Inport  Port=5
  KeSMSuFoldType : Inport  Port=6
  unfold3LAvl : Inport  Port=7
  unfold3RAvl : Inport  Port=8
  PassCmprtMdHMIReqExt : Inport  Port=9
  StPassCmprtMdHMIReqExt2 : Inport  Port=10
  StPassUnfold3LReq : Inport  Port=11
  StPassCmprtMdCtrl_Md32_VCUConfig : Inport  Port=12
  StPassCmprtMdCtrl_Md53_VCUConfig : Inport  Port=13
  StSrv_StMd32_Config : Inport  Port=14
  AND{,1..6} (7 alike) : Logic  AllPortsSameDT=off  OutDataTypeStr=boolean
  ButtonLongPressed : Subsystem  AncestorBlock=MSMLib/ButtonLongPressed
  ButtonLongPressed1 : Subsystem  AncestorBlock=MSMLib/ButtonLongPressed
  ConfirmRequireSource : MSMLib/ConfirmRequireSource  SystemSampleTime=-1
  ConfirmRequireSource1 : MSMLib/ConfirmRequireSource  SystemSampleTime=-1
  Constant : Constant  Value=0  OutDataTypeStr=boolean
  Constant1 : Constant  Value=10  OutDataTypeStr=uint8
  Constant19 : Constant  Value=9  OutDataTypeStr=uint8
  Constant2 : Constant  Value=CmprtMdHMIReqExtTp1.CmprtMdHMIReqExtTp_Mode32  OutDataTypeStr=Enum:CmprtMdHMIReqExtTp1
  Constant3 : Constant  Value=CmprtMdHMIReqExtTp1.CmprtMdHMIReqExtTp_NoAction  OutDataTypeStr=Enum:CmprtMdHMIReqExtTp1
  Constant4 : Constant  Value=CmprtMdHMIReqExt2Tp1.CmprtMdHMIReqExt2Tp_Mode53  OutDataTypeStr=Enum:CmprtMdHMIReqExt2Tp1
  Constant5 : Constant  Value=CmprtMdHMIReqExt2Tp1.CmprtMdHMIReqExt2Tp_NoAction  OutDataTypeStr=Enum:CmprtMdHMIReqExt2Tp1
  Constant6 : Constant  Value=true  OutDataTypeStr=boolean
  Constant7 : Constant  Value=0  OutDataTypeStr=boolean
  Constant8 : Constant  Value=0  OutDataTypeStr=boolean
  Equal1 : RelationalOperator  Operator=~=  OutDataTypeStr=boolean  RndMeth=Simplest
  Equal17 : RelationalOperator  Operator=~=  OutDataTypeStr=boolean  RndMeth=Simplest
  Equal2 : RelationalOperator  Operator===  OutDataTypeStr=boolean  RndMeth=Simplest
  Equal3 : RelationalOperator  Operator===  OutDataTypeStr=boolean  RndMeth=Simplest
  Equal4 : RelationalOperator  Operator===  OutDataTypeStr=boolean  RndMeth=Simplest
  Equal5 : RelationalOperator  Operator=~=  OutDataTypeStr=boolean  RndMeth=Simplest
  Ground : Ground
  Ground1 : Ground
  Logical Operator : Logic  Operator=OR  Inputs=3  AllPortsSameDT=off  OutDataTypeStr=boolean
  Logical Operator1 : Logic  Operator=OR  AllPortsSameDT=off  OutDataTypeStr=boolean
  Logical Operator2 : Logic  Operator=OR  AllPortsSameDT=off  OutDataTypeStr=boolean
  NOT : Logic  Operator=NOT  AllPortsSameDT=off  OutDataTypeStr=boolean
  NOT1 : Logic  Operator=NOT  AllPortsSameDT=off  OutDataTypeStr=boolean
  Relational Operator1 : RelationalOperator  Operator===  OutDataTypeStr=boolean  RndMeth=Simplest
  Relational Operator3 : RelationalOperator  Operator===  OutDataTypeStr=boolean  RndMeth=Simplest
  SWIntSrc_S : MSMLib/SWIntSrc_S  SystemSampleTime=-1
  SWIntSrc_S1 : MSMLib/SWIntSrc_S  SystemSampleTime=-1
  Subsystem1 : MSMLib/MergeReqAndValidity  SystemSampleTime=-1
  Subsystem4 : MSMLib/MergeReqAndValidity  SystemSampleTime=-1
  Switch{,1..6} (7 alike) : Switch  Criteria=u2 > Threshold
  Unit Delay{,1..2,5..7,19} (7 alike) : UnitDelay  SampleTime=-1
  Unit Delay3 : UnitDelay  InitialCondition=g  SampleTime=-1
  Unit Delay4 : UnitDelay  InitialCondition=j  SampleTime=-1
  SwUnfold3LIntCnt : Outport
  SwUnfold3RIntCnt : Outport  Port=2
  Unfold3LReq : Outport  Port=3  VectorParamsAs1DForOutWhenUnconnected=on
  Unfold3LsrcReqTp : Outport  Port=4  VectorParamsAs1DForOutWhenUnconnected=on
  Unfold3LNotf1ChimeEventStat : Outport  Port=5
  Unfold3RReq : Outport  Port=6  VectorParamsAs1DForOutWhenUnconnected=on
  Unfold3RsrcReqTp : Outport  Port=7  VectorParamsAs1DForOutWhenUnconnected=on
  Unfold3RNotf1ChimeEventStat : Outport  Port=8
  Unfold3LSoftInt : Outport  Port=9
  Unfold3RSoftInt : Outport  Port=10
  wires:
  Constant19/1 -> SWIntSrc_S/2
  ButtonLongPressed/2(mdInterruptCnt) -> SwUnfold3LIntCnt/1, Unit Delay19/1, Equal17/1
  Unit Delay19/1 -> Equal17/2
  Subsystem4/1 -> ButtonLongPressed/1(modeReq)
  ThdRLtStExpdSwReqV/1 -> Subsystem4/2
  Equal17/1 -> SWIntSrc_S/1
  ThdRLtStExpdSwReq/1 -> Subsystem4/1
  buttonLongPressedThrshhldTm/1 -> [buttonLongPressedThrshhldTm]
  [buttonLongPressedThrshhldTm] -> ButtonLongPressed/2(longPressThrshhldTm)
  ThdRRtStExpdSwReq/1 -> Subsystem1/1
  ThdRRtStExpdSwReqV/1 -> Subsystem1/2
  Subsystem1/1 -> ButtonLongPressed1/1(modeReq)
  Equal1/1 -> SWIntSrc_S1/1
  Unit Delay1/1 -> Equal1/2
  Constant1/1 -> SWIntSrc_S1/2
  ButtonLongPressed1/2(mdInterruptCnt) -> SwUnfold3RIntCnt/1, Unit Delay1/1, Equal1/1
  [buttonLongPressedThrshhldTm] -> ButtonLongPressed1/2(longPressThrshhldTm)
  unfold3LAvl/1 -> Switch3/2, Switch1/2, NOT/1
  NOT/1 -> AND/2
  Unit Delay/1 -> Switch1/3
  AND/1 -> Unfold3LNotf1ChimeEventStat/1
  ConfirmRequireSource/1 -> Unfold3LsrcReqTp/1
  Switch1/1 -> Unit Delay/1, Unfold3LReq/1
  Ground/1 -> ConfirmRequireSource/6, ConfirmRequireSource/3, ConfirmRequireSource/2
  ButtonLongPressed/1(mdReq) -> AND1/2
  KeSMSuFoldType/1 -> [KeSMSuFoldType]
  [KeSMSuFoldType] -> AND1/1
  AND1/1 -> [SwUnfold3LMdReq]
  ButtonLongPressed1/1(mdReq) -> AND2/2
  AND2/1 -> [SwUnfold3RMdReq]
  [KeSMSuFoldType] -> AND2/1
  Ground1/1 -> ConfirmRequireSource1/2, ConfirmRequireSource1/3, ConfirmRequireSource1/6, ConfirmRequireSource1/5
  Switch2/1 -> Unfold3RReq/1, Unit Delay2/1
  ConfirmRequireSource1/1 -> Unfold3RsrcReqTp/1
  AND3/1 -> Unfold3RNotf1ChimeEventStat/1
  Unit Delay2/1 -> Switch2/3
  NOT1/1 -> AND3/2
  unfold3RAvl/1 -> Switch4/2, NOT1/1, Switch2/2
  Equal2/1 -> AND5/2
  Constant2/1 -> Relational Operator3/2
  Unit Delay3/1 -> Equal2/1
  PassCmprtMdHMIReqExt/1 -> Relational Operator3/1, Unit Delay3/1
  Constant3/1 -> Equal2/2
  Relational Operator3/1 -> AND5/1
  StPassCmprtMdHMIReqExt2/1 -> Unit Delay4/1, Relational Operator1/1
  Constant4/1 -> Relational Operator1/2
  Unit Delay4/1 -> Equal3/1
  Constant5/1 -> Equal3/2
  Relational Operator1/1 -> AND4/1
  Equal3/1 -> AND4/2
  Switch3/1 -> Unit Delay5/1, Unfold3LSoftInt/1
  Unit Delay5/1 -> Switch3/3
  Switch4/1 -> Unit Delay6/1, Unfold3RSoftInt/1
  Unit Delay6/1 -> Switch4/3
  Unit Delay7/1 -> Equal5/1
  Equal4/1 -> AND6/1
  Equal5/1 -> AND6/2
  Constant6/1 -> Equal5/2, Equal4/2
  StPassUnfold3LReq/1 -> Unit Delay7/1, Equal4/1
  [SwUnfold3LMdReq] -> ConfirmRequireSource/1, Logical Operator/1
  [passCmprtMdHMIReq_unfold3L] -> ConfirmRequireSource/4, Logical Operator1/2, Logical Operator/3
  [Unfold3LReq] -> ConfirmRequireSource/5, Logical Operator1/1, Logical Operator/2
  Logical Operator/1 -> Switch1/1, AND/1
  Logical Operator1/1 -> Switch3/1
  [SwUnfold3RMdReq] -> ConfirmRequireSource1/1, Logical Operator2/1
  [passCmprtMdHMIReq_unfold3R] -> ConfirmRequireSource1/4, Switch4/1, Logical Operator2/2
  Logical Operator2/1 -> Switch2/1, AND3/1
  StPassCmprtMdCtrl_Md32_VCUConfig/1 -> Switch/2
  AND5/1 -> Switch/1
  Constant/1 -> Switch/3
  Switch/1 -> [passCmprtMdHMIReq_unfold3L]
  AND4/1 -> Switch5/1
  StPassCmprtMdCtrl_Md53_VCUConfig/1 -> Switch5/2
  Constant7/1 -> Switch5/3
  Switch5/1 -> [passCmprtMdHMIReq_unfold3R]
  AND6/1 -> Switch6/1
  StSrv_StMd32_Config/1 -> Switch6/2
  Constant8/1 -> Switch6/3
  Switch6/1 -> [Unfold3LReq]

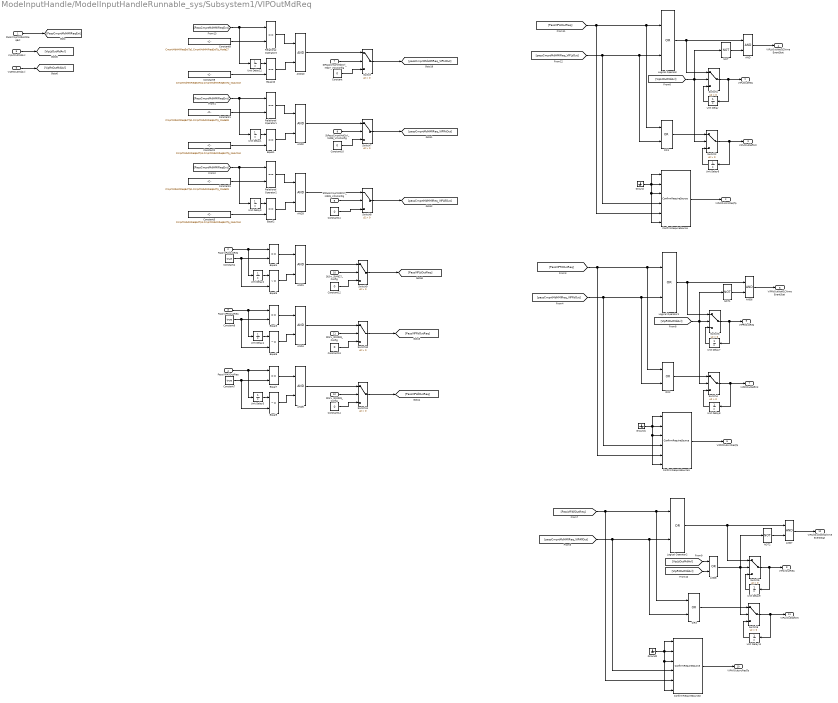
== system ModeInputHandle/ModelInputHandleRunnable_sys/Subsystem1/VIPOutMdReq ==
  PassCmprtMdHMIReqExt : Inport
  PassVIPLtOutReq : Inport  Port=2
  PassVIPRtOutReq : Inport  Port=3
  PassVIPAllOutReq : Inport  Port=4
  VipLtOutMdAvl : Inport  Port=5
  VipRtOutMdAvl : Inport  Port=6
  StPassCmprtMdCtrl_Md27_VCUConfig : Inport  Port=7
  StPassCmprtMdCtrl_Md28_VCUConfig : Inport  Port=8
  StPassCmprtMdCtrl_Md29_VCUConfig : Inport  Port=9
  StSrv_StMd27_Config : Inport  Port=10
  StSrv_StMd28_Config : Inport  Port=11
  StSrv_StMd29_Config : Inport  Port=12
  AND{,1..7,10} (9 alike) : Logic  AllPortsSameDT=off  OutDataTypeStr=boolean
  AND8 : Logic  Operator=OR  AllPortsSameDT=off  OutDataTypeStr=boolean
  ConfirmRequireSource : MSMLib/ConfirmRequireSource  SystemSampleTime=-1
  ConfirmRequireSource1 : MSMLib/ConfirmRequireSource  SystemSampleTime=-1
  ConfirmRequireSource2 : MSMLib/ConfirmRequireSource  SystemSampleTime=-1
  Constant{,10..14} (6 alike) : Constant  Value=0  OutDataTypeStr=boolean
  Constant1 : Constant  Value=CmprtMdHMIReqExtTp1.CmprtMdHMIReqExtTp_Mode28  OutDataTypeStr=Enum:CmprtMdHMIReqExtTp1
  Constant2 : Constant  Value=CmprtMdHMIReqExtTp1.CmprtMdHMIReqExtTp_NoAction  OutDataTypeStr=Enum:CmprtMdHMIReqExtTp1
  Constant3 : Constant  Value=CmprtMdHMIReqExtTp1.CmprtMdHMIReqExtTp_Mode29  OutDataTypeStr=Enum:CmprtMdHMIReqExtTp1
  Constant4 : Constant  Value=true  OutDataTypeStr=boolean
  Constant5 : Constant  Value=CmprtMdHMIReqExtTp1.CmprtMdHMIReqExtTp_NoAction  OutDataTypeStr=Enum:CmprtMdHMIReqExtTp1
  Constant6 : Constant  Value=true  OutDataTypeStr=boolean
  Constant7 : Constant  Value=true  OutDataTypeStr=boolean
  Constant8 : Constant  Value=CmprtMdHMIReqExtTp1.CmprtMdHMIReqExtTp_Mode27  OutDataTypeStr=Enum:CmprtMdHMIReqExtTp1
  Constant9 : Constant  Value=CmprtMdHMIReqExtTp1.CmprtMdHMIReqExtTp_NoAction  OutDataTypeStr=Enum:CmprtMdHMIReqExtTp1
  Equal{1..4,7,10} (6 alike) : RelationalOperator  Operator===  OutDataTypeStr=boolean  RndMeth=Simplest
  Equal5 : RelationalOperator  Operator=~=  OutDataTypeStr=boolean  RndMeth=Simplest
  Equal6 : RelationalOperator  Operator=~=  OutDataTypeStr=boolean  RndMeth=Simplest
  Equal9 : RelationalOperator  Operator=~=  OutDataTypeStr=boolean  RndMeth=Simplest
  Ground : Ground
  Ground1 : Ground
  Ground2 : Ground
  Logical Operator : Logic  Operator=OR  AllPortsSameDT=off  OutDataTypeStr=boolean
  Logical Operator1 : Logic  Operator=OR  AllPortsSameDT=off  OutDataTypeStr=boolean
  Logical Operator2 : Logic  Operator=OR  AllPortsSameDT=off  OutDataTypeStr=boolean
  NOT : Logic  Operator=NOT  AllPortsSameDT=off  OutDataTypeStr=boolean
  NOT1 : Logic  Operator=NOT  AllPortsSameDT=off  OutDataTypeStr=boolean
  NOT2 : Logic  Operator=NOT  AllPortsSameDT=off  OutDataTypeStr=boolean
  OR1 : Logic  Operator=OR  AllPortsSameDT=off  OutDataTypeStr=boolean
  OR2 : Logic  Operator=OR  AllPortsSameDT=off  OutDataTypeStr=boolean
  OR3 : Logic  Operator=OR  AllPortsSameDT=off  OutDataTypeStr=boolean
  Relational Operator1 : RelationalOperator  Operator===  OutDataTypeStr=boolean  RndMeth=Simplest
  Relational Operator2 : RelationalOperator  Operator===  OutDataTypeStr=boolean  RndMeth=Simplest
  Relational Operator3 : RelationalOperator  Operator===  OutDataTypeStr=boolean  RndMeth=Simplest
  Switch{,1..11} (12 alike) : Switch  Criteria=u2 > Threshold
  Unit Delay{,2,4..9,11} (9 alike) : UnitDelay  SampleTime=-1
  Unit Delay1 : UnitDelay  InitialCondition=g  SampleTime=-1
  Unit Delay12 : UnitDelay  InitialCondition=g  SampleTime=-1
  Unit Delay3 : UnitDelay  InitialCondition=g  SampleTime=-1
  VIPLtOutReq : Outport  VectorParamsAs1DForOutWhenUnconnected=on
  VIPLtOutsrcReqTp : Outport  Port=2  VectorParamsAs1DForOutWhenUnconnected=on
  VIPLtOutSoftInt : Outport  Port=3
  VIPLtOutNotf1ChimeEventStat : Outport  Port=4
  VIPRtOutReq : Outport  Port=5  VectorParamsAs1DForOutWhenUnconnected=on
  VIPRtOutsrcReqTp : Outport  Port=6  VectorParamsAs1DForOutWhenUnconnected=on
  VIPRtOutSoftInt : Outport  Port=7
  VIPRtOutNotf1ChimeEventStat : Outport  Port=8
  VIPAllOutReq : Outport  Port=9  VectorParamsAs1DForOutWhenUnconnected=on
  VIPAllOutsrcReqTp : Outport  Port=10  VectorParamsAs1DForOutWhenUnconnected=on
  VIPAllOutSoftInt : Outport  Port=11
  VIPAllOutNotf1ChimeEventStat : Outport  Port=12
  wires:
  Equal4/1 -> AND1/1
  Equal5/1 -> AND1/2
  PassVIPLtOutReq/1 -> Equal4/1, Unit Delay2/1
  Constant4/1 -> Equal5/2, Equal4/2
  Unit Delay2/1 -> Equal5/1
  Unit Delay4/1 -> Equal6/1
  Constant6/1 -> Equal3/2, Equal6/2
  PassVIPRtOutReq/1 -> Unit Delay4/1, Equal3/1
  Equal6/1 -> AND4/2
  Equal3/1 -> AND4/1
  Equal7/1 -> AND5/1
  Equal9/1 -> AND5/2
  PassVIPAllOutReq/1 -> Equal7/1, Unit Delay5/1
  Constant7/1 -> Equal9/2, Equal7/2
  Unit Delay5/1 -> Equal9/1
  NOT/1 -> AND/2
  OR1/1 -> Switch2/1
  Switch2/1 -> VIPLtOutSoftInt/1, Unit Delay6/1
  Unit Delay/1 -> Switch1/3
  Unit Delay6/1 -> Switch2/3
  Logical Operator/1 -> Switch1/1, AND/1
  AND/1 -> VIPLtOutNotf1ChimeEventStat/1
  ConfirmRequireSource/1 -> VIPLtOutsrcReqTp/1
  [passCmprtMdHMIReq_VIPLtOut] -> ConfirmRequireSource/4, OR1/2, Logical Operator/2
  [PassVIPLtOutReq] -> ConfirmRequireSource/5, OR1/1, Logical Operator/1
  Switch1/1 -> Unit Delay/1, VIPLtOutReq/1
  Ground/1 -> ConfirmRequireSource/1, ConfirmRequireSource/6, ConfirmRequireSource/3, ConfirmRequireSource/2
  Ground1/1 -> ConfirmRequireSource1/2, ConfirmRequireSource1/3, ConfirmRequireSource1/6, ConfirmRequireSource1/1
  Switch3/1 -> VIPRtOutReq/1, Unit Delay7/1
  [PassVIPRtOutReq] -> Logical Operator1/1, OR2/1, ConfirmRequireSource1/5
  [passCmprtMdHMIReq_VIPRtOut] -> Logical Operator1/2, OR2/2, ConfirmRequireSource1/4
  ConfirmRequireSource1/1 -> VIPRtOutsrcReqTp/1
  AND6/1 -> VIPRtOutNotf1ChimeEventStat/1
  Logical Operator1/1 -> AND6/1, Switch3/1
  Unit Delay8/1 -> Switch4/3
  Unit Delay7/1 -> Switch3/3
  Switch4/1 -> Unit Delay8/1, VIPRtOutSoftInt/1
  OR2/1 -> Switch4/1
  NOT1/1 -> AND6/2
  AND8/1 -> Switch6/2, NOT2/1, Switch5/2
  NOT2/1 -> AND7/2
  OR3/1 -> Switch6/1
  Switch6/1 -> VIPAllOutSoftInt/1, Unit Delay11/1
  Unit Delay9/1 -> Switch5/3
  Unit Delay11/1 -> Switch6/3
  Logical Operator2/1 -> Switch5/1, AND7/1
  AND7/1 -> VIPAllOutNotf1ChimeEventStat/1
  ConfirmRequireSource2/1 -> VIPAllOutsrcReqTp/1
  [passCmprtMdHMIReq_VIPAllOut] -> ConfirmRequireSource2/4, OR3/2, Logical Operator2/2
  [PassVIPAllOutReq] -> ConfirmRequireSource2/5, OR3/1, Logical Operator2/1
  Switch5/1 -> Unit Delay9/1, VIPAllOutReq/1
  Ground2/1 -> ConfirmRequireSource2/1, ConfirmRequireSource2/6, ConfirmRequireSource2/3, ConfirmRequireSource2/2
  VipLtOutMdAvl/1 -> [VipLtOutMdAvl]
  [VipLtOutMdAvl] -> Switch2/2, NOT/1, Switch1/2
  VipRtOutMdAvl/1 -> [VipRtOutMdAvl]
  [VipRtOutMdAvl] -> Switch4/2, NOT1/1, Switch3/2
  [VipLtOutMdAvl] -> AND8/1
  [VipRtOutMdAvl] -> AND8/2
  Constant8/1 -> Relational Operator3/2
  Constant9/1 -> Equal10/2
  Equal10/1 -> AND10/2
  Relational Operator3/1 -> AND10/1
  Unit Delay12/1 -> Equal10/1
  PassCmprtMdHMIReqExt/1 -> [PassCmprtMdHMIReqExt]
  [PassCmprtMdHMIReqExt] -> Unit Delay12/1, Relational Operator3/1
  [PassCmprtMdHMIReqExt] -> Relational Operator1/1, Unit Delay1/1
  Unit Delay1/1 -> Equal1/1
  Relational Operator1/1 -> AND2/1
  Equal1/1 -> AND2/2
  Constant2/1 -> Equal1/2
  Constant1/1 -> Relational Operator1/2
  Constant3/1 -> Relational Operator2/2
  Constant5/1 -> Equal2/2
  Equal2/1 -> AND3/2
  Relational Operator2/1 -> AND3/1
  Unit Delay3/1 -> Equal2/1
  [PassCmprtMdHMIReqExt] -> Unit Delay3/1, Relational Operator2/1
  StPassCmprtMdCtrl_Md27_VCUConfig/1 -> Switch/2
  Switch/1 -> [passCmprtMdHMIReq_VIPLtOut]
  AND10/1 -> Switch/1
  Constant/1 -> Switch/3
  AND2/1 -> Switch7/1
  StPassCmprtMdCtrl_Md28_VCUConfig/1 -> Switch7/2
  Constant10/1 -> Switch7/3
  Switch7/1 -> [passCmprtMdHMIReq_VIPRtOut]
  AND3/1 -> Switch8/1
  Switch8/1 -> [passCmprtMdHMIReq_VIPAllOut]
  StPassCmprtMdCtrl_Md29_VCUConfig/1 -> Switch8/2
  Constant11/1 -> Switch8/3
  AND1/1 -> Switch9/1
  StSrv_StMd27_Config/1 -> Switch9/2
  Constant12/1 -> Switch9/3
  Switch9/1 -> [PassVIPLtOutReq]
  AND4/1 -> Switch10/1
  StSrv_StMd28_Config/1 -> Switch10/2
  Constant13/1 -> Switch10/3
  Switch10/1 -> [PassVIPRtOutReq]
  AND5/1 -> Switch11/1
  StSrv_StMd29_Config/1 -> Switch11/2
  Switch11/1 -> [PassVIPAllOutReq]
  Constant14/1 -> Switch11/3
